simulink model "quad_altitude"  (R2026a)
settings: Solver=ode3  StopTime=12  FixedStep=0.001
PreLoadFcn:
  | P = quad_params();
libraries: slpidlib x1
settings Model: Creator=Vismay  LastModifiedBy=Vismay

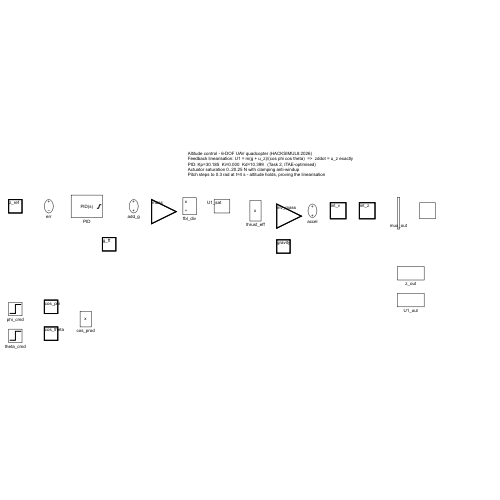
[thumbnail: Simulink's stored preview of the top-level diagram]
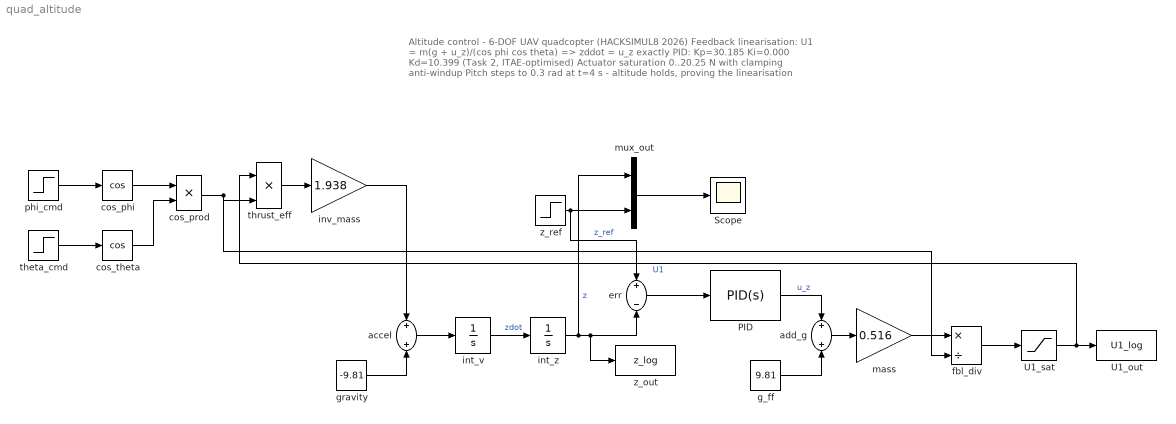
== system quad_altitude ==
  note: Altitude control - 6-DOF UAV quadcopter (HACKSIMUL8 2026)
      | Feedback linearisation: U1 = m(g + u_z)/(cos phi cos theta)  =>  zddot = u_z exactly
      | PID: Kp=30.185  Ki=0.000  Kd=10.399   (Task 2, ITAE-optimised)
      | Actuator saturation 0..20.25 N with clamping anti-windup
      | Pitch steps to 0.3 rad at t=4 s - altitude holds, proving the linearisation
  PID : slpidlib/PID Controller  Controller=PID  Form=Parallel  TimeDomain=Continuous-time  UseExternalTs=off  SampleTime=-1  IntegratorMethod=Forward Euler  FilterMethod=Forward Euler  ControllerParametersSource=internal  P=30.1847  I=7.8503e-07  UseKiTs=off  D=10.3994  UseExternalDerivativeSource=off  N=100  UseFilter=on  TunerSelectOption=Transfer Function Based (PID Tuner App)  InitialConditionSource=internal  InitialConditionForIntegrator=0  InitialConditionForFilter=0  DifferentiatorICPrevScaledInput=0  ExternalReset=none  TrackingMode=off  Kt=1  LimitOutput=on  SatLimitsSource=internal  UpperSaturationLimit=39.24  LowerSaturationLimit=-9.81  LinearizeAsGain=on  AntiWindupMode=clamping  Kb=1  LimitIntegrator=off  UpperIntegratorSaturationLimit=inf  LowerIntegratorSaturationLimit=-inf  POutMin=[]  POutMax=[]  IOutMin=[]  IOutMax=[]  DOutMin=[]  DOutMax=[]  NOutMin=[]  NOutMax=[]  SumOutMin=[]  SumOutMax=[]  SaturationOutMin=[]  SaturationOutMax=[]  PParamMin=[]  PParamMax=[]  IParamMin=[]  IParamMax=[]  DParamMin=[]  DParamMax=[]  NParamMin=[]  NParamMax=[]  KbParamMin=[]  KbParamMax=[]  KtParamMin=[]  KtParamMax=[]  KbOutMin=[]  KbOutMax=[]  KtOutMin=[]  KtOutMax=[]  IntegratorOutMin=[]  IntegratorOutMax=[]  FilterOutMin=[]  FilterOutMax=[]  SumI1OutMin=[]  SumI1OutMax=[]  SumI2OutMin=[]  SumI2OutMax=[]  SumI3OutMin=[]  SumI3OutMax=[]  SumI4OutMin=[]  SumI4OutMax=[]  SumDOutMin=[]  SumDOutMax=[]  DifferentiatorOutMin=[]  DifferentiatorOutMax=[]  FilterDiffOutCoefMin=[]  FilterDiffOutCoefMax=[]  ReciprocalOutMin=[]  ReciprocalOutMax=[]  SumDenOutMin=[]  SumDenOutMax=[]  SumNumOutMin=[]  SumNumOutMax=[]  DivideOutMin=[]  DivideOutMax=[]  UdiffTsProdOutMin=[]  UdiffTsProdOutMax=[]  NTsProdOutMin=[]  NTsProdOutMax=[]  UintegralTsProdOutMin=[]  UintegralTsProdOutMax=[]  UngainTsProdOutMin=[]  UngainTsProdOutMax=[]  ClampingZeroOutDataTypeStr=Inherit: Inherit via back propagation  ClampingZeroOutMin=[]  ClampingZeroOutMax=[]  FilterDenConstantOutDataTypeStr=Inherit: Inherit via back propagation  FilterDenConstantOutMin=[]  FilterDenConstantOutMax=[]  PCopyOutDataTypeStr=Inherit: Inherit via back propagation  PCopyOutMin=[]  PCopyOutMax=[]  NCopyOutDataTypeStr=Inherit: Inherit via back propagation  NCopyOutMin=[]  NCopyOutMax=[]  IntegratorContinuousStateAttributes=''  IntegratorStateMustResolveToSignalObject=off  IntegratorRTWStateStorageClass=Auto  FilterContinuousStateAttributes=''  FilterStateMustResolveToSignalObject=off  FilterRTWStateStorageClass=Auto  ParallelPVariant=InternalParameters  IdealPVariant=Disabled  IVariant=InternalParameters  DVariant=InternalParameters  IntegratorVariant=Continuous  SatVariant=Enabled  AWVariant=ContClampingParallel  PCopyVariant=Disabled  TRVariant=Disabled  FdbkBlocksVariant=Forward  IdealPFdbkVariant=Disabled  SatFdbkVariant=Disabled  DerivativeFilterVariant=ContFilter  NVariant=InternalParameters  NCopyVariant=Disabled  FilterICVariant=InternalICsFilter  IntegratorICVariant=InternalICs  ExternalResetVariant=Disabled  TRSumVariant=Passthrough  SumFdbkVariant=Disabled  SumVariant=Sum_PID  TsampFilterVariant=InternalTs  TsampNgainVariant=Passthrough  TsampIntegralVariant=Disabled_SignalSpec  ExternalSaturationOutDataTypeStr=Inherit: Same as second input  DerivativeSourceVariant=ErrorSignal  PreIntVariant=InternalPreInt
  Scope : Scope
  U1_out : ToWorkspace  VariableName=U1_log  SaveFormat=Structure With Time  SampleTime=-1
  U1_sat : Saturate  UpperLimit=20.2478  LowerLimit=0
  accel : Sum
  add_g : Sum
  cos_phi : Trigonometry  Operator=cos
  cos_prod : Product
  cos_theta : Trigonometry  Operator=cos
  err : Sum  Inputs=+-
  fbl_div : Product  Inputs=*/
  g_ff : Constant  Value=9.81
  gravity : Constant  Value=-9.81
  int_v : Integrator
  int_z : Integrator
  inv_mass : Gain  Gain=1.938
  mass : Gain  Gain=0.516
  mux_out : Mux  Inputs=2
  phi_cmd : Step  Time=100  FinalValue=0  SampleTime=0
  theta_cmd : Step  Time=4  FinalValue=0.3  SampleTime=0
  thrust_eff : Product
  z_out : ToWorkspace  VariableName=z_log  SaveFormat=Structure With Time  SampleTime=-1
  z_ref : Step  SampleTime=0
  wires:
  cos_phi/1 -> cos_prod/1
  phi_cmd/1 -> cos_phi/1
  thrust_eff/1 -> inv_mass/1
  theta_cmd/1 -> cos_theta/1
  cos_prod/1 -> thrust_eff/2, fbl_div/2
  cos_theta/1 -> cos_prod/2
  inv_mass/1 -> accel/1
  gravity/1 -> accel/2
  accel/1 -> int_v/1
  int_v/1 -> int_z/1  "zdot"
  fbl_div/1 -> U1_sat/1
  z_ref/1 -> err/1, mux_out/2  "z_ref"
  int_z/1 -> z_out/1, err/2, mux_out/1  "z"
  mux_out/1 -> Scope/1
  err/1 -> PID/1
  mass/1 -> fbl_div/1
  PID/1 -> add_g/1  "u_z"
  g_ff/1 -> add_g/2
  add_g/1 -> mass/1
  U1_sat/1 -> U1_out/1, thrust_eff/1  "U1"
